simulink model "SIM_EXO_DAL"  (R2021b)
settings: Solver=VariableStepAuto  StartTime=0.0  StopTime=60  FixedStep=0.0001  RelTol=1e-4
undefined symbols (not defined in the file): b, dq, q, X, Y, Z
libraries: sm_lib x47, nesl_utility x7
(part 8 of 25)

== matlab function SIM_EXO_DAL/Exoesqueleto/Dinámica Directa/MATLAB Function3 ==
  data: H input; He output
function He = He(H)
    j=8.0790e-10;

    J=j*eye(6);

    n=1;

    N=n*eye(6);

    He=H+J*N^2;

end

== matlab function SIM_EXO_DAL/MATLAB Function ==
  data: tau input; P output; dq input
function P = Potencia(tau,dq)
    P = zeros(6,1);
    for i = 1:6
        P(i) = tau(i)*dq(i);
    end
